simulink subsystem "Position_PI_D"  (R2022b)
settings: Solver=VariableStepAuto  StartTime=0.0  StopTime=10.0  RelTol=1e-3
undefined symbols (not defined in the file or in its folder): conv, DiscIntNeverNeededParam, Ri, Rt, Rw, sat, uc
settings Model: Creator=gotta  LastModifiedBy=berti

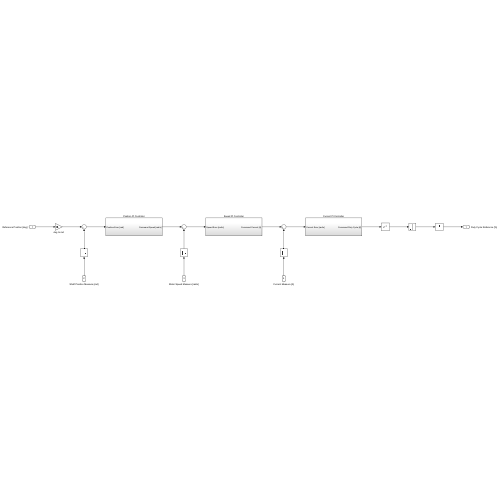
[thumbnail: Simulink's stored preview of the top-level diagram]
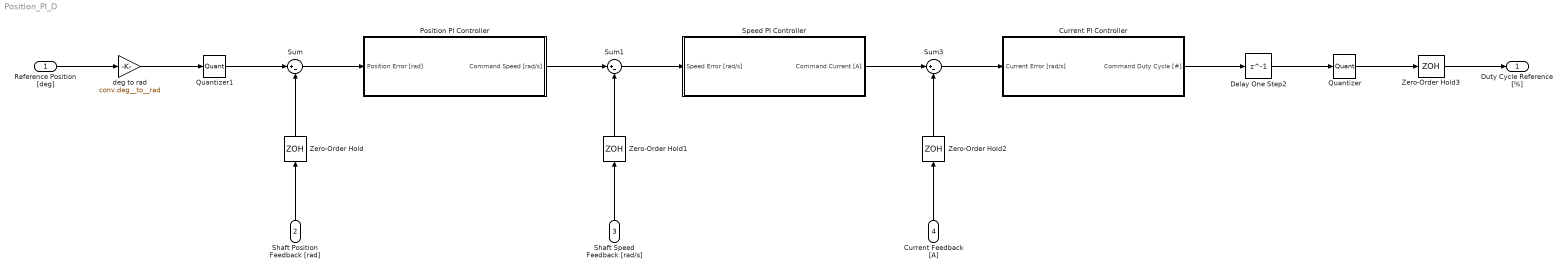
== system Position_PI_D ==
  Reference Position [deg] : Inport
  Shaft Position Feedback [rad] : Inport  Port=2
  Shaft Speed Feedback [rad/s] : Inport  Port=3
  Current Feedback [A] : Inport  Port=4
  Current PI Controller : Subsystem
  Delay One Step2 : Delay  DelayLength=1
  Position PI Controller : Subsystem
  Quantizer : Quantizer  QuantizationInterval=uc.d_step
  Quantizer1 : Quantizer  QuantizationInterval=AS5600.q_rad
  Speed PI Controller : Subsystem
  Sum : Sum  Inputs=|+-
  Sum1 : Sum  Inputs=|+-
  Sum3 : Sum  Inputs=|+-
  Zero-Order Hold{,1..3} (4 alike) : ZeroOrderHold  SampleTime=uc.Ts
  deg to rad : Gain  Gain=conv.deg__to__rad
  Duty Cycle Reference [%] : Outport
  wires:
  Sum1/1 -> Speed PI Controller/1(Speed Error [rad/s])
  Quantizer/1 -> Zero-Order Hold3/1
  Reference Position [deg]/1 -> deg to rad/1
  Current Feedback [A]/1 -> Zero-Order Hold2/1
  Shaft Speed Feedback [rad/s]/1 -> Zero-Order Hold1/1
  Speed PI Controller/1(Command Current [A]) -> Sum3/1
  Sum3/1 -> Current PI Controller/1(Current Error [rad/s])
  Current PI Controller/1(Command Duty Cycle [#]) -> Delay One Step2/1
  Shaft Position Feedback [rad]/1 -> Zero-Order Hold/1
  Position PI Controller/1(Command Speed [rad/s]) -> Sum1/1
  deg to rad/1 -> Quantizer1/1
  Delay One Step2/1 -> Quantizer/1
  Zero-Order Hold/1 -> Sum/2
  Zero-Order Hold1/1 -> Sum1/2
  Zero-Order Hold2/1 -> Sum3/2
  Sum/1 -> Position PI Controller/1(Position Error [rad])
  Zero-Order Hold3/1 -> Duty Cycle Reference [%]/1
  Quantizer1/1 -> Sum/1

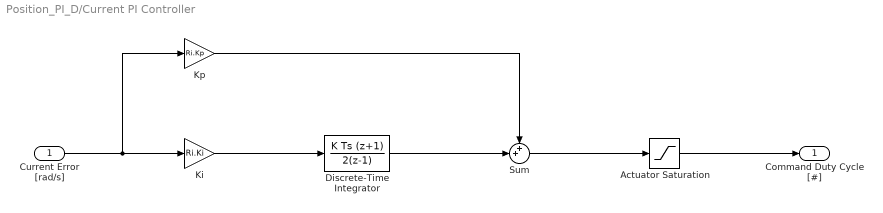
== system Position_PI_D/Current PI Controller ==
  Current Error [rad/s] : Inport
  Actuator Saturation : Saturate  UpperLimit=sat.d  LowerLimit=-sat.d
  Discrete-Time Integrator : DiscreteIntegrator  IntegratorMethod=Integration: Trapezoidal  SampleTime=uc.Ts  LimitOutput=on  UpperSaturationLimit=sat.d/2  LowerSaturationLimit=-sat.d/2  ICPrevOutput=DiscIntNeverNeededParam  ICPrevScaledInput=DiscIntNeverNeededParam
  Ki : Gain  Gain=Ri.Ki
  Kp : Gain  Gain=Ri.Kp
  Sum : Sum  Inputs=++|
  Command Duty Cycle [#] : Outport
  wires:
  Actuator Saturation/1 -> Command Duty Cycle [#]/1
  Current Error [rad/s]/1 -> Kp/1, Ki/1
  Kp/1 -> Sum/1
  Sum/1 -> Actuator Saturation/1
  Ki/1 -> Discrete-Time Integrator/1
  Discrete-Time Integrator/1 -> Sum/2

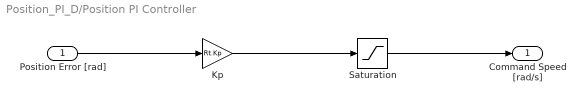
== system Position_PI_D/Position PI Controller ==
  Position Error [rad] : Inport
  Kp : Gain  Gain=Rt.Kp
  Saturation : Saturate  UpperLimit=sat.w  LowerLimit=-sat.w
  Command Speed [rad/s] : Outport
  wires:
  Kp/1 -> Saturation/1
  Position Error [rad]/1 -> Kp/1
  Saturation/1 -> Command Speed [rad/s]/1

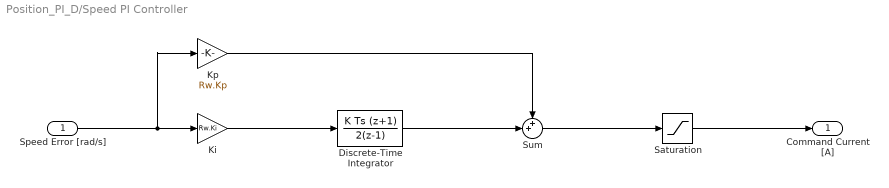
== system Position_PI_D/Speed PI Controller ==
  Speed Error [rad/s] : Inport
  Discrete-Time Integrator : DiscreteIntegrator  IntegratorMethod=Integration: Trapezoidal  SampleTime=uc.Ts  LimitOutput=on  UpperSaturationLimit=sat.I/2  LowerSaturationLimit=-sat.I/2  ICPrevOutput=DiscIntNeverNeededParam  ICPrevScaledInput=DiscIntNeverNeededParam
  Ki : Gain  Gain=Rw.Ki
  Kp : Gain  Gain=Rw.Kp
  Saturation : Saturate  UpperLimit=sat.I  LowerLimit=-sat.I
  Sum : Sum  Inputs=++|
  Command Current [A] : Outport
  wires:
  Kp/1 -> Sum/1
  Saturation/1 -> Command Current [A]/1
  Speed Error [rad/s]/1 -> Ki/1, Kp/1
  Sum/1 -> Saturation/1
  Ki/1 -> Discrete-Time Integrator/1
  Discrete-Time Integrator/1 -> Sum/2
